simulink model "airspeed"  (R2018a)
settings: Solver=FixedStepAuto  StartTime=0.0  StopTime=10.0  FixedStep=0.001  RelTol=1e-3
undefined symbols (not defined in the file): magnitude
libraries: simulink_extras x1
settings Model: Creator=David  LastModifiedBy=David

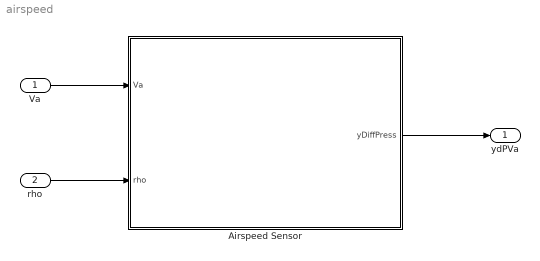
== system airspeed ==
  Va : Inport
  rho : Inport  Port=2
  Airspeed Sensor : Subsystem  mask{SampleTime=1, diffPressureNoiseDensity=0, diffPressureBandwidthHz=1E06, diffPressureInit=0, diffPressureUpperSaturation=inf, diffPressureLowerSaturation=-inf, diffPressureResolution=1E-12}
      mask prompts: SampleTime "Airspeed Sensor Sample Time (s)"; diffPressureNoiseDensity "Airspeed Pressure Sensor Noise Density (Pa/sqrt(Hz))"; diffPressureBandwidthHz "Airspeed Pressure Sensor Bandwidth (Hz)"; diffPressureInit "Airspeed Pressure Sensor Initial Condition (Pa)"; diffPressureUpperSaturation "Airspeed Pressure Sensor Upper Saturation Limit (Pa)"; diffPressureLowerSaturation "Airspeed Pressure Sensor Lower Saturation Limit (Pa)"; diffPressureResolution "Airspeed Pressure Sensor Resolution (Pa)"
      mask DialogControl DescGroupVar Prompt: Pitot Tube Airspeed Sensor Model
      mask DialogControl DescTextVar Prompt: Pitot Tube Airspeed Sensor with White Noise Modelling.
      mask DialogControl Control2 Prompt: If one can only get a sensor accuracy of +- error band of span, treat this as 3 sigma when calculating noise density. (ie. ((Sensor % Band)/3)*Span/(sqrt(1/SamplingTime))
      mask DialogControl Container7 Prompt: System Characteristics
      mask DialogControl Container4 Prompt: Noise Characteristics
      mask DialogControl Container6 Prompt: Sensor Dynamics
      mask DialogControl Container10 Prompt: Bandwidth
      mask DialogControl Container11 Prompt: Initial Conditions
      mask DialogControl Container8 Prompt: Limits and Quantization
      mask DialogControl Container13 Prompt: Limits
      mask DialogControl Container16 Prompt: Quantization
      mask Display:
      | image('airspeed_sensor.jpg')
      | 
      | color('red')
      | 
      | port_label('input', 1, 'V_a (m/s)', 'texMode', 'on')
      | port_label('input', 2, '\rho (kg/m^3)', 'texMode', 'on')
      | 
      | port_label('output', 1, 'y_{\DeltaP_{V_a}} (Pa)', 'texMode', 'on')
  ydPVa : Outport
  wires:
  Va/1 -> Airspeed Sensor/1(Va)
  Airspeed Sensor/1(yDiffPress) -> ydPVa/1
  rho/1 -> Airspeed Sensor/2(rho)

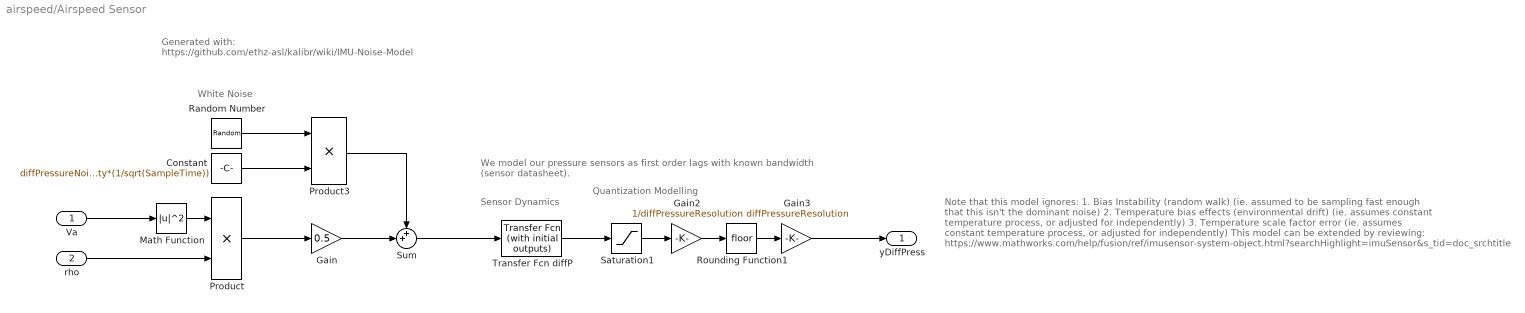
== system airspeed/Airspeed Sensor ==
  note: White Noise
  note: Generated with:
      | https://github.com/ethz-asl/kalibr/wiki/IMU-Noise-Model
  note: We model our pressure sensors as first order lags with known bandwidth
      | (sensor datasheet).
  note: Sensor Dynamics
  note: Quantization Modelling
  note: Note that this model ignores:
      | 1. Bias Instability (random walk) (ie. assumed to be sampling fast enough that this isn't the dominant noise)
      | 2. Temperature bias effects (environmental drift) (ie. assumes constant temperature process, or adjusted for independently)
      | 3. Temperature scale factor error (ie. assumes constant temperature process, or adjusted for independently)
      |
      | This model can be extended by reviewing:
      | https://www.mathworks.com/help/fusion/ref/imusensor-system-object.html?searchHighlight=imuSensor&s_tid=doc_srchtitle
  Va : Inport
  rho : Inport  Port=2
  Constant : Constant  Value=diffPressureNoiseDensity*(1/sqrt(SampleTime))
  Gain : Gain  Gain=0.5
  Gain2 : Gain  Gain=1/diffPressureResolution
  Gain3 : Gain  Gain=diffPressureResolution
  Math Function : Math  Operator=magnitude^2  SaturateOnIntegerOverflow=on
  Product : Product
  Product3 : Product
  Random Number : RandomNumber  SampleTime=SampleTime
  Rounding Function1 : Rounding
  Saturation1 : Saturate  UpperLimit=diffPressureUpperSaturation  LowerLimit=diffPressureLowerSaturation
  Sum : Sum  Inputs=++|
  Transfer Fcn diffP : simulink_extras/Additional Linear/Transfer Fcn (with initial outputs)  N=[diffPressureBandwidthHz*2*pi]  D="[1,  diffPressureBandwidthHz*2*pi]"  Y0=diffPressureInit  U0=diffPressureInit
  yDiffPress : Outport
  wires:
  Va/1 -> Math Function/1
  Random Number/1 -> Product3/1
  Product3/1 -> Sum/1
  Constant/1 -> Product3/2
  Math Function/1 -> Product/1
  rho/1 -> Product/2
  Product/1 -> Gain/1
  Gain/1 -> Sum/2
  Transfer Fcn diffP/1 -> Saturation1/1
  Sum/1 -> Transfer Fcn diffP/1
  Gain2/1 -> Rounding Function1/1
  Saturation1/1 -> Gain2/1
  Gain3/1 -> yDiffPress/1
  Rounding Function1/1 -> Gain3/1
